simulink subsystem "kinematics"  (R2024b)
settings: Solver=VariableStepAuto  StartTime=0.0  StopTime=10.0  RelTol=1e-3
undefined symbols (not defined in the file): DiscIntNeverNeededParam
settings Model: Creator=yagiz  LastModifiedBy=yagiz

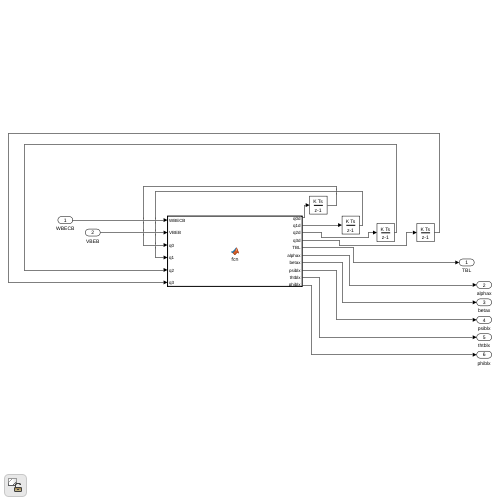
[thumbnail: Simulink's stored preview of the top-level diagram]
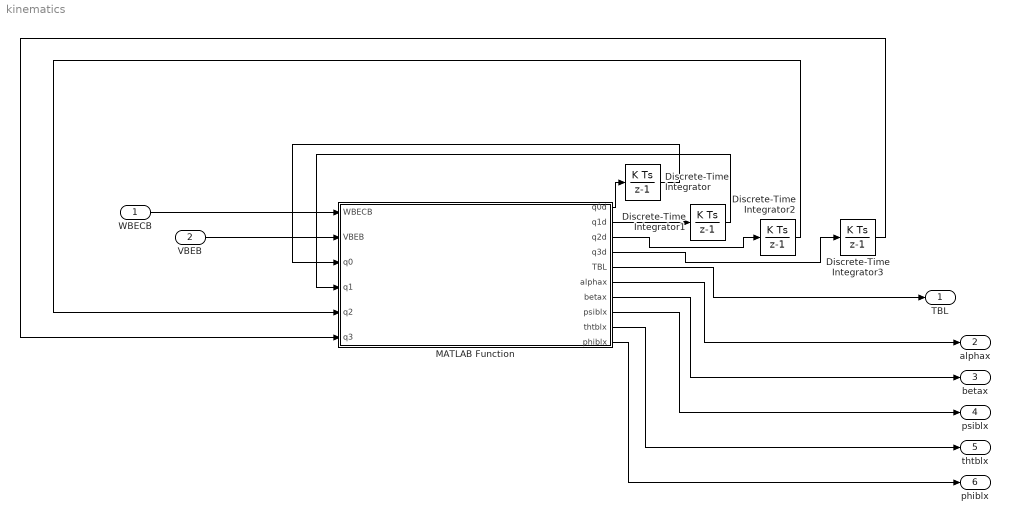
== system kinematics ==
  WBECB : Inport
  VBEB : Inport  Port=2
  Discrete-Time Integrator : DiscreteIntegrator  InitialCondition=1  SampleTime=0.001  ICPrevOutput=DiscIntNeverNeededParam  ICPrevScaledInput=DiscIntNeverNeededParam
  Discrete-Time Integrator1 : DiscreteIntegrator  SampleTime=0.001  ICPrevOutput=DiscIntNeverNeededParam  ICPrevScaledInput=DiscIntNeverNeededParam
  Discrete-Time Integrator2 : DiscreteIntegrator  SampleTime=0.001  ICPrevOutput=DiscIntNeverNeededParam  ICPrevScaledInput=DiscIntNeverNeededParam
  Discrete-Time Integrator3 : DiscreteIntegrator  SampleTime=0.001  ICPrevOutput=DiscIntNeverNeededParam  ICPrevScaledInput=DiscIntNeverNeededParam
  MATLAB Function : MATLAB Function  TreatAsAtomicUnit=on
  TBL : Outport
  alphax : Outport  Port=2
  betax : Outport  Port=3
  psiblx : Outport  Port=4
  thtblx : Outport  Port=5
  phiblx : Outport  Port=6
  wires:
  WBECB/1 -> MATLAB Function/1(WBECB)
  VBEB/1 -> MATLAB Function/2(VBEB)
  MATLAB Function/1(q0d) -> Discrete-Time Integrator/1
  MATLAB Function/2(q1d) -> Discrete-Time Integrator1/1
  Discrete-Time Integrator/1 -> MATLAB Function/3(q0)
  Discrete-Time Integrator1/1 -> MATLAB Function/4(q1)
  MATLAB Function/3(q2d) -> Discrete-Time Integrator2/1
  Discrete-Time Integrator2/1 -> MATLAB Function/5(q2)
  MATLAB Function/4(q3d) -> Discrete-Time Integrator3/1
  Discrete-Time Integrator3/1 -> MATLAB Function/6(q3)
  MATLAB Function/5(TBL) -> TBL/1
  MATLAB Function/6(alphax) -> alphax/1
  MATLAB Function/7(betax) -> betax/1
  MATLAB Function/8(psiblx) -> psiblx/1
  MATLAB Function/9(thtblx) -> thtblx/1
  MATLAB Function/10(phiblx) -> phiblx/1

== matlab function kinematics/MATLAB Function ==
  data: WBECB input; q0d output; VBEB input; q0 input; q1 input; q2 input; q3 input; q1d output; q2d output; q3d output; TBL output; alphax output; betax output; psiblx output; thtblx output; phiblx output
function [q0d,q1d,q2d,q3d,TBL,alphax,betax,psiblx,thtblx,phiblx] = fcn(WBECB,VBEB,q0,q1,q2,q3)

pp = WBECB(1); qq = WBECB(2); rr = WBECB(3);
ck = 50.0; EPS = 1e-10; DEG = 180/pi;

% Quaternion derivatives (with orthogonality correction)
oe  = 1.0 - (q0^2 + q1^2 + q2^2 + q3^2);
q0d = 0.5*(-pp*q1 - qq*q2 - rr*q3) + ck*oe*q0;
q1d = 0.5*( pp*q0 + rr*q2 - qq*q3) + ck*oe*q1;
q2d = 0.5*( qq*q0 - rr*q1 + pp*q3) + ck*oe*q2;
q3d = 0.5*( rr*q0 + qq*q1 - pp*q2) + ck*oe*q3;

% DCM from quaternion
TBL = [q0^2+q1^2-q2^2-q3^2,  2*(q1*q2+q0*q3),         2*(q1*q3-q0*q2);
       2*(q1*q2-q0*q3),        q0^2-q1^2+q2^2-q3^2,    2*(q2*q3+q0*q1);
       2*(q1*q3+q0*q2),        2*(q2*q3-q0*q1),          q0^2-q1^2-q2^2+q3^2];

% Euler angles from DCM
tbl13 = TBL(1,3);
if abs(tbl13) < 1.0
    thtbl  = asin(-tbl13);
    cthtbl = cos(thtbl);
else
    thtbl  = sign(-tbl13)*pi/2;
    cthtbl = EPS;
end
cpsi = max(-1+EPS, min(1-EPS, TBL(1,1)/cthtbl));
cphi = max(-1+EPS, min(1-EPS, TBL(3,3)/cthtbl));
psiblx = sign(TBL(1,2)) * acos(cpsi) * DEG;
thtblx = thtbl * DEG;
phiblx = sign(TBL(2,3)) * acos(cphi) * DEG;

% Incidence angles from body velocity
vb1 = VBEB(1); vb2 = VBEB(2); vb3 = VBEB(3);
dvbe = max(sqrt(vb1^2+vb2^2+vb3^2), EPS);
alphax = atan2(vb3, vb1) * DEG;
betax  = asin(max(-1.0, min(1.0, vb2/dvbe))) * DEG;
